simulink model "StateEstimatorComplete"  (R2022a)
settings: Solver=ode4  StartTime=0.0  StopTime=200  FixedStep=0.1  RelTol=1e-3
values from neighbouring files (symbols this model uses):
  A = [1.0034,0.0207,0.4737,0.0463,-0.2364,2.3069;    -0.0011,0.9997,-0.0541,0.1380,0.9540,-13.3772;     0.0000,0.0000,0.9424,0.6183,-0.2177,2.1255;    -0.0000,-0.0000,0.1676,-0.8000,0.4213,-5.1737;     0.0000,-0.0002,-0.0060,0.1014,-0.1223,-12.4611;    -0.0000,0.0000,-0.0000,-0.0004,-0.0028,-0.5637]    [Kalman_initializing.m]
  B = 1.0e-08 *[-0.8484,-0.3258,-0.1868;     0.4781,-0.1277,-0.2667;    -0.0948,-0.0255,-0.0254;     0.2341,0.0767,0.1066;    -0.0197,-0.0031,-0.1006;    -0.0005,-0.0006,0.0006]    [Kalman_initializing.m]
  C = [0.6830,-0.1854,-0.2271,0.6690,0.0090,0.0006 ... (first row only)    [Kalman_initializing.m]
  D = 1.0e-08 *[-0.3458,-0.1652,-0.0717;    -0.0376,-0.0129,-0.1373;     0.0011,0.0020,-0.0003]    [Kalman_initializing.m]
  K = [34.8690,9.8057,11.2373;   -20.4980,36.9942,21.6928;     4.6280,-0.6726,-33.1105;   -12.2170,-0.1861,-5.2135;    -3.8993,12.7559,16.9157;     0.0335,-0.0487,-11.0087]    [Kalman_initializing.m]
libraries: dspsrcs4 x3, realtime_pacer_lib x1
settings Model: Creator=Jan-Robin  LastModifiedBy=Jan-Robin

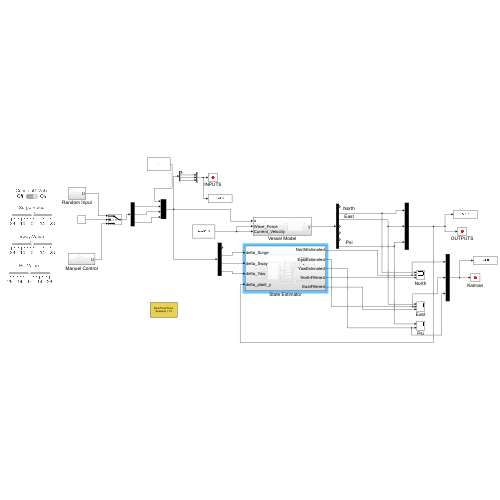
[thumbnail: Simulink's stored preview of the top-level diagram]
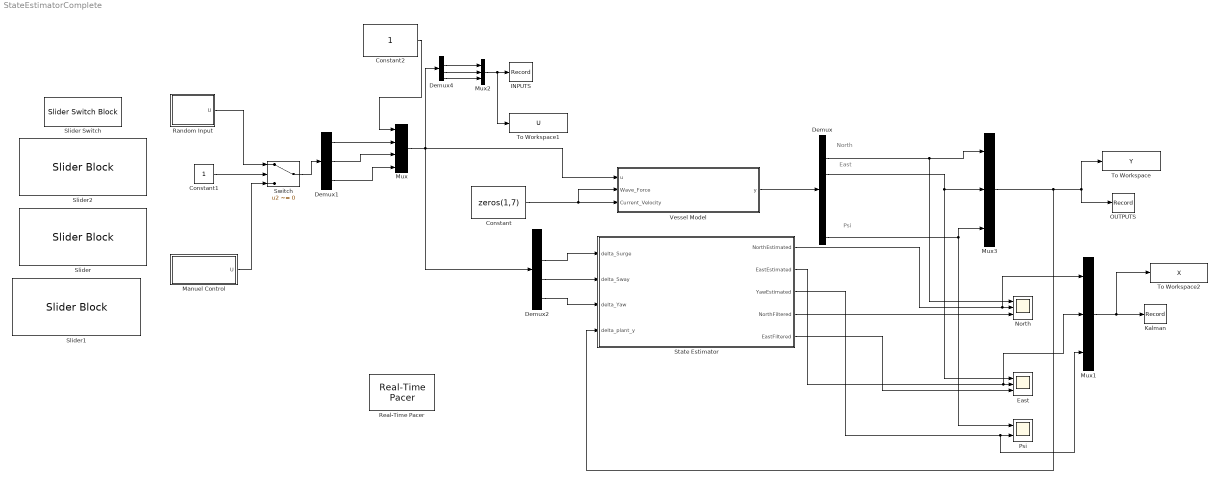
== system StateEstimatorComplete ==
  note: Psi
  note: East
  note: North
  Constant : Constant  Value=zeros(1,7)
  Constant1 : Constant
  Constant2 : Constant
  Demux : Demux  Outputs=7
  Demux1 : Demux  Outputs=3
  Demux2 : Demux
  Demux4 : Demux
  East : Scope  NumInputPorts=3
  INPUTS : Record  VariableName=INPUT  RecordToWorkspace=on  FileSettingsInternal="{\"entries\":[{\"content\":{\"excelSettings\":{\"content\":{},\"type\":\"Streamout.ExcelSettings\"}},\"type\":\"Streamout.FileSettingStorage\",\"uuid\":\"\"}],\"packageUris\":[\"http:\\/\\/schema.mathworks.com\\/mf0\\/streamout_blocks\\/R2020a\"],\"version\":\"1.0\"}"  SignalsInternal="{\"entries\":[{\"content\":{\"signals\":[{\"content\":{\"blockPath\":[],\"channel\":[],\"dimensions\":[3],\"domain\":\"\",\"hasChildren\":true,\"lineColor\":\"#ff6929\",\"plots\":[],\"port\":1,\"sid\":[\"\"],\"signalID\":6521,\"signalName\":\"Mux2\"},\"type\":\"RecordBlkView.Signal\",\"uuid\":\"\"},{\"content\":{\"blockPath\":[],\"channel\":[1],\"dimensions\":[3],\"domain\":\"\",\"lineColor\":\"#ff6929\",\"parentID\":6521,\"plots\":[1],\"port\":1,\"sid\":[\"\"],\"signalID\":6522,\"signalName\":\"Mux2\"},\"type\":\"RecordBlkView.Signal\",\"uuid\":\"\"},{\"content\":{\"blockPath\":[],\"channel\":[2],\"dimensions\":[3],\"domain\":\"\",\"lineColor\":\"#b746ff\",\"parentID\":6521,\"plots\":[1],\"port\":1,\"sid\":[\"\"],\"signalID\":6588,\"signalName\":\"Mux2\"},\"type\":\"RecordBlkView.Signal\",\"uuid\":\"\"},{\"content\":{\"blockPath\":[],\"channel\":[3],\"dimensions\":[3],\"domain\":\"\",\"lineColor\":\"#64d413\",\"parentID\":6521,\"plots\":[1],\"port\":1,\"sid\":[\"\"],\"signalID\":6589,\"signalName\":\"Mux2\"},\"type\":\"RecordBlkView.Signal\",\"uuid\":\"\"}]},\"type\":\"RecordBlkView.InputSignals\",\"uuid\":\"\"}],\"packageUris\":[\"http:\\/\\/schema.mathworks.com\\/mf0\\/streamout_blocks\\/R2020a\"],\"version\":\"1.0\"}"  VisualizationBindings="{\"sparklinesplugin\":{\"info\":[{\"bindingParametersList\":[],\"subplotID\":1}]}}"
  Kalman : Record  VariableName=KALMAN  RecordToWorkspace=on  FileSettingsInternal="{\"entries\":[{\"content\":{\"excelSettings\":{\"content\":{},\"type\":\"Streamout.ExcelSettings\"}},\"type\":\"Streamout.FileSettingStorage\",\"uuid\":\"\"}],\"packageUris\":[\"http:\\/\\/schema.mathworks.com\\/mf0\\/streamout_blocks\\/R2020a\"],\"version\":\"1.0\"}"  Layout=[1 1]  SignalsInternal="{\"entries\":[{\"content\":{\"signals\":[{\"content\":{\"blockPath\":[],\"channel\":[],\"dimensions\":[3],\"domain\":\"\",\"hasChildren\":true,\"lineColor\":\"#64d413\",\"plots\":[],\"port\":1,\"sid\":[\"\"],\"signalID\":6526,\"signalName\":\"Mux1\"},\"type\":\"RecordBlkView.Signal\",\"uuid\":\"\"},{\"content\":{\"blockPath\":[],\"channel\":[1],\"dimensions\":[3],\"domain\":\"\",\"lineColor\":\"#139fff\",\"parentID\":6526,\"plots\":[],\"port\":1,\"sid\":[\"\"],\"signalID\":6527,\"signalName\":\"Mux1\"},\"type\":\"RecordBlkView.Signal\",\"uuid\":\"\"},{\"content\":{\"blockPath\":[],\"channel\":[2],\"dimensions\":[3],\"domain\":\"\",\"lineColor\":\"#7e2f8e\",\"parentID\":6526,\"plots\":[],\"port\":1,\"sid\":[\"\"],\"signalID\":6590,\"signalName\":\"Mux1\"},\"type\":\"RecordBlkView.Signal\",\"uuid\":\"\"},{\"content\":{\"blockPath\":[],\"channel\":[3],\"dimensions\":[3],\"domain\":\"\",\"lineColor\":\"#77ac30\",\"parentID\":6526,\"plots\":[],\"port\":1,\"sid\":[\"\"],\"signalID\":6591,\"signalName\":\"Mux1\"},\"type\":\"RecordBlkView.Signal\",\"uuid\":\"\"}]},\"type\":\"RecordBlkView.InputSignals\",\"uuid\":\"\"}],\"packageUris\":[\"http:\\/\\/schema.mathworks.com\\/mf0\\/streamout_blocks\\/R2020a\"],\"version\":\"1.0\"}"  VisualizationBindings="{\"sparklinesplugin\":{\"info\":[{\"bindingParametersList\":[],\"subplotID\":1}]}}"
  Manuel Control : Subsystem
  Mux : Mux
  Mux1 : Mux  Inputs=3
  Mux2 : Mux  Inputs=3
  Mux3 : Mux  Inputs=3
  North : Scope  NumInputPorts=3
  OUTPUTS : Record  VariableName=OUTPUT  RecordToWorkspace=on  FileSettingsInternal="{\"entries\":[{\"content\":{\"excelSettings\":{\"content\":{},\"type\":\"Streamout.ExcelSettings\"}},\"type\":\"Streamout.FileSettingStorage\",\"uuid\":\"\"}],\"packageUris\":[\"http:\\/\\/schema.mathworks.com\\/mf0\\/streamout_blocks\\/R2020a\"],\"version\":\"1.0\"}"  Layout=[1 1]  SignalsInternal="{\"entries\":[{\"content\":{\"signals\":[{\"content\":{\"blockPath\":[],\"channel\":[],\"dimensions\":[3],\"domain\":\"\",\"hasChildren\":true,\"lineColor\":\"#fe330a\",\"plots\":[],\"port\":1,\"sid\":[\"\"],\"signalID\":6531,\"signalName\":\"Mux3\"},\"type\":\"RecordBlkView.Signal\",\"uuid\":\"\"},{\"content\":{\"blockPath\":[],\"channel\":[1],\"dimensions\":[3],\"domain\":\"\",\"lineColor\":\"#b746ff\",\"parentID\":6531,\"plots\":[],\"port\":1,\"sid\":[\"\"],\"signalID\":6532,\"signalName\":\"Mux3\"},\"type\":\"RecordBlkView.Signal\",\"uuid\":\"\"},{\"content\":{\"blockPath\":[],\"channel\":[2],\"dimensions\":[3],\"domain\":\"\",\"lineColor\":\"#4dbeee\",\"parentID\":6531,\"plots\":[],\"port\":1,\"sid\":[\"\"],\"signalID\":6592,\"signalName\":\"Mux3\"},\"type\":\"RecordBlkView.Signal\",\"uuid\":\"\"},{\"content\":{\"blockPath\":[],\"channel\":[3],\"dimensions\":[3],\"domain\":\"\",\"lineColor\":\"#a2142f\",\"parentID\":6531,\"plots\":[],\"port\":1,\"sid\":[\"\"],\"signalID\":6593,\"signalName\":\"Mux3\"},\"type\":\"RecordBlkView.Signal\",\"uuid\":\"\"}]},\"type\":\"RecordBlkView.InputSignals\",\"uuid\":\"\"}],\"packageUris\":[\"http:\\/\\/schema.mathworks.com\\/mf0\\/streamout_blocks\\/R2020a\"],\"version\":\"1.0\"}"  VisualizationBindings="{\"sparklinesplugin\":{\"info\":[{\"bindingParametersList\":[],\"subplotID\":1}]}}"
  Psi : Scope  NumInputPorts=2
  Random Input : Subsystem
  Real-Time Pacer : realtime_pacer_lib/Real-Time Pacer  simTimePerRealTime=10
      settings: SourceProductName=Real-Time Pacer
  Slider : SliderBlock  ScaleMin=-28  ScaleMax=28
  Slider Switch : SliderSwitchBlock
      settings: Values={{'Off', 'On'}, [0 1]}
  Slider1 : SliderBlock  ScaleMin=-28  ScaleMax=28
  Slider2 : SliderBlock  ScaleMin=-28  ScaleMax=28
  State Estimator : Subsystem
  Switch : Switch  Criteria=u2 ~= 0  SaturateOnIntegerOverflow=off  InputSameDT=off
  To Workspace : ToWorkspace  VariableName=Y  SampleTime=0.1
  To Workspace1 : ToWorkspace  VariableName=U  SampleTime=0.1
  To Workspace2 : ToWorkspace  VariableName=X  SampleTime=0.1
  Vessel Model : Subsystem
  wires:
  Demux4/3 -> Mux2/2
  Demux4/2 -> Mux2/1
  Demux4/4 -> Mux2/3
  Constant2/1 -> Mux/1
  Vessel Model/1(y) -> Demux/1
  Mux/1 -> Demux2/1, Vessel Model/1(u), Demux4/1
  Mux2/1 -> To Workspace1/1, INPUTS/1
  Demux/7 -> Psi/1, Mux3/3
  Constant/1 -> Vessel Model/2(Wave_Force), Vessel Model/3(Current_Velocity)
  Mux3/1 -> OUTPUTS/1, To Workspace/1, State Estimator/4(delta_plant_y)
  Demux2/2 -> State Estimator/1(delta_Surge)
  Demux2/3 -> State Estimator/2(delta_Sway)
  Demux2/4 -> State Estimator/3(delta_Yaw)
  Demux/2 -> Mux3/1, North/1
  State Estimator/1(NorthEstimated) -> Mux1/1, North/2
  State Estimator/2(EastEstimated) -> Mux1/2, East/2
  State Estimator/3(YawEstimated) -> Mux1/3, Psi/2
  State Estimator/4(NorthFiltered) -> North/3
  State Estimator/5(EastFiltered) -> East/3
  Mux1/1 -> To Workspace2/1, Kalman/1
  Demux/3 -> Mux3/2, East/1
  Random Input/1(U) -> Switch/1
  Constant1/1 -> Switch/2
  Manuel Control/1(U) -> Switch/3
  Switch/1 -> Demux1/1
  Demux1/1 -> Mux/2
  Demux1/2 -> Mux/3
  Demux1/3 -> Mux/4

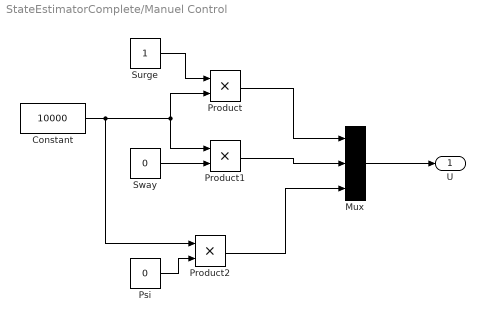
== system StateEstimatorComplete/Manuel Control ==
  Constant : Constant  Value=10000
  Mux : Mux  Inputs=3
  Product : Product
  Product1 : Product
  Product2 : Product
  Psi : Constant  Value=0
  Surge : Constant
  Sway : Constant  Value=0
  U : Outport
  wires:
  Mux/1 -> U/1
  Surge/1 -> Product/1
  Constant/1 -> Product2/1, Product/2, Product1/1
  Sway/1 -> Product1/2
  Psi/1 -> Product2/2
  Product2/1 -> Mux/3
  Product1/1 -> Mux/2
  Product/1 -> Mux/1

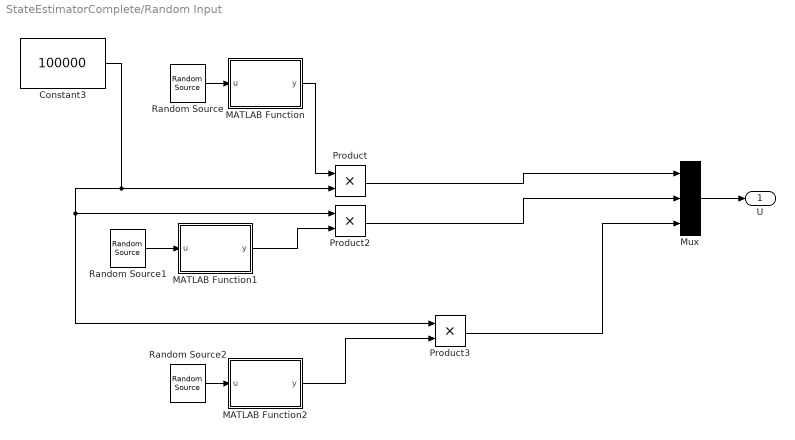
== system StateEstimatorComplete/Random Input ==
  Constant3 : Constant  Value=100000
  MATLAB Function : MATLAB Function  TreatAsAtomicUnit=on
  MATLAB Function1 : MATLAB Function  TreatAsAtomicUnit=on
  MATLAB Function2 : MATLAB Function  TreatAsAtomicUnit=on
  Mux : Mux  Inputs=3
  Product : Product
  Product2 : Product
  Product3 : Product
  Random Source : dspsrcs4/Random Source  SrcType=Uniform  NormMethod=Ziggurat  CltLength=12  MinVal=-1  MaxVal=1  MeanVal=0  VarVal=1  RepMode=Not repeatable  rawSeed=1  IsInherit=off  SampMode=Continuous  SampTime=10  SampFrame=1  DataType=Single  OutComplex=Real  OutputFrames=off
  Random Source1 : dspsrcs4/Random Source  SrcType=Uniform  NormMethod=Ziggurat  CltLength=12  MinVal=-1  MaxVal=1  MeanVal=0  VarVal=1  RepMode=Not repeatable  rawSeed=1  IsInherit=off  SampMode=Continuous  SampTime=10  SampFrame=1  DataType=Single  OutComplex=Real  OutputFrames=off
  Random Source2 : dspsrcs4/Random Source  SrcType=Uniform  NormMethod=Ziggurat  CltLength=12  MinVal=-1  MaxVal=1  MeanVal=0  VarVal=1  RepMode=Not repeatable  rawSeed=1  IsInherit=off  SampMode=Continuous  SampTime=10  SampFrame=1  DataType=Single  OutComplex=Real  OutputFrames=off
  U : Outport
  wires:
  Random Source1/1 -> MATLAB Function1/1(u)
  Constant3/1 -> Product/2, Product2/1, Product3/1
  MATLAB Function1/1(y) -> Product2/2
  Random Source2/1 -> MATLAB Function2/1(u)
  Product2/1 -> Mux/2
  Product/1 -> Mux/1
  Random Source/1 -> MATLAB Function/1(u)
  MATLAB Function2/1(y) -> Product3/2
  MATLAB Function/1(y) -> Product/1
  Product3/1 -> Mux/3
  Mux/1 -> U/1

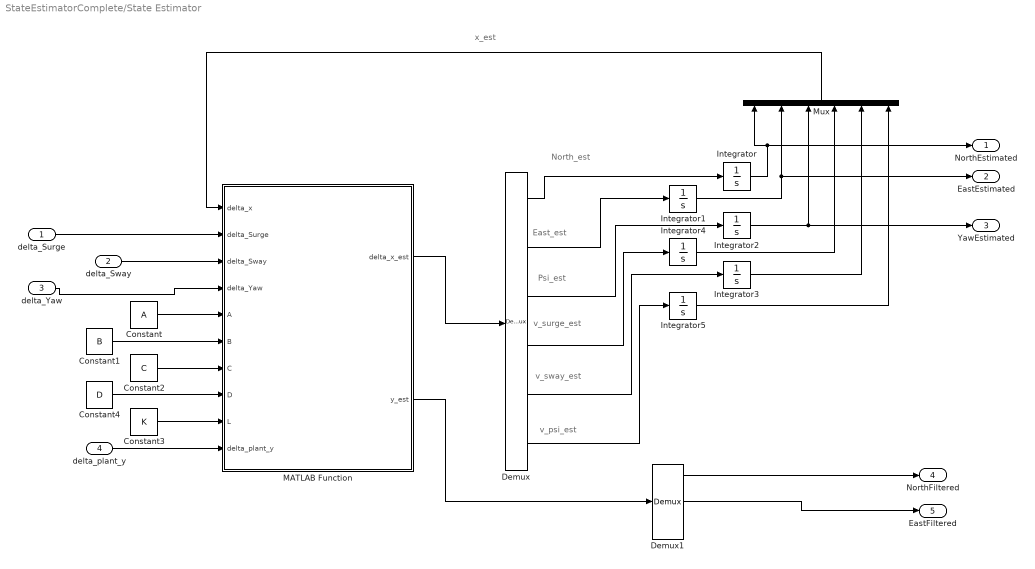
== system StateEstimatorComplete/State Estimator ==
  note: x_est
  note: v_psi_est
  note: v_sway_est
  note: v_surge_est
  note: Psi_est
  note: East_est
  note: North_est
  delta_Surge : Inport
  delta_Sway : Inport  Port=2
  delta_Yaw : Inport  Port=3
  delta_plant_y : Inport  Port=4
  Constant : Constant  Value=A
  Constant1 : Constant  Value=B
  Constant2 : Constant  Value=C
  Constant3 : Constant  Value=K
  Constant4 : Constant  Value=D
  Demux : Demux  Outputs=6
  Demux1 : Demux  Outputs=3
  Integrator : Integrator  LimitOutput=on  UpperSaturationLimit=100  LowerSaturationLimit=-100
  Integrator1 : Integrator  LimitOutput=on  UpperSaturationLimit=100  LowerSaturationLimit=-100
  Integrator2 : Integrator  InitialCondition=-0.0005  UpperSaturationLimit=0.02  LowerSaturationLimit=-0.02
  Integrator3 : Integrator  InitialCondition=0.0067  LimitOutput=on  UpperSaturationLimit=4  LowerSaturationLimit=-4
  Integrator4 : Integrator  InitialCondition=0.1385  LimitOutput=on  UpperSaturationLimit=4  LowerSaturationLimit=-4
  Integrator5 : Integrator  InitialCondition=-0.0017  LimitOutput=on  UpperSaturationLimit=0.2  LowerSaturationLimit=-0.2
  MATLAB Function : MATLAB Function  TreatAsAtomicUnit=on
  Mux : Mux  Inputs=6
  NorthEstimated : Outport
  EastEstimated : Outport  Port=2
  YawEstimated : Outport  Port=3
  NorthFiltered : Outport  Port=4
  EastFiltered : Outport  Port=5
  wires:
  delta_Surge/1 -> MATLAB Function/2(delta_Surge)
  delta_Sway/1 -> MATLAB Function/3(delta_Sway)
  delta_Yaw/1 -> MATLAB Function/4(delta_Yaw)
  delta_plant_y/1 -> MATLAB Function/10(delta_plant_y)
  Constant2/1 -> MATLAB Function/7(C)
  Constant3/1 -> MATLAB Function/9(L)
  MATLAB Function/1(delta_x_est) -> Demux/1
  Demux/1 -> Integrator/1
  Demux/2 -> Integrator1/1
  Demux/3 -> Integrator2/1
  Demux/4 -> Integrator4/1
  Demux/5 -> Integrator3/1
  Demux/6 -> Integrator5/1
  Integrator/1 -> Mux/1, NorthEstimated/1
  Integrator1/1 -> EastEstimated/1, Mux/2
  Integrator2/1 -> YawEstimated/1, Mux/3
  Integrator4/1 -> Mux/4
  Integrator3/1 -> Mux/5
  Integrator5/1 -> Mux/6
  Constant/1 -> MATLAB Function/5(A)
  Constant1/1 -> MATLAB Function/6(B)
  Constant4/1 -> MATLAB Function/8(D)
  Mux/1 -> MATLAB Function/1(delta_x)
  MATLAB Function/2(y_est) -> Demux1/1
  Demux1/1 -> NorthFiltered/1
  Demux1/2 -> EastFiltered/1

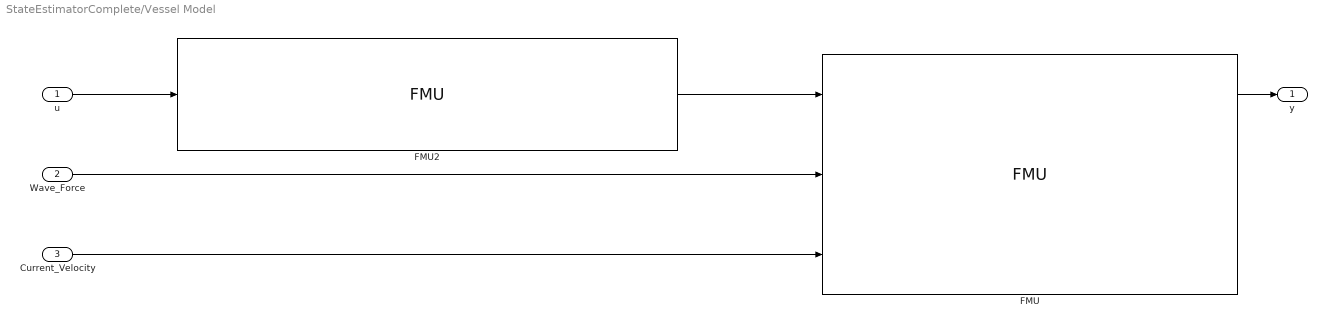
== system StateEstimatorComplete/Vessel Model ==
  u : Inport
  Wave_Force : Inport  Port=2
  Current_Velocity : Inport  Port=3
  FMU : FMU  FMUName=VesselModel.fmu  FMUMode=CoSimulation  Axc=106.0  Ayc=419.0  Bv_0_=44000.0  Bv_1_=0.0  Bv_2_=0.0  Bv_3_=0.0  Bv_4_=0.0  Bv_5_=0.0  Bv_6_=0.0  Bv_7_=177000.0  Bv_8_=0.0  Bv_9_=0.0  Bv_10_=0.0  Bv_11_=0.0  Bv_12_=0.0  Bv_13_=0.0  Bv_14_=0.0  Bv_15_=0.0  Bv_16_=0.0  Bv_17_=0.0  Bv_18_=0.0  Bv_19_=0.0  Bv_20_=0.0  Bv_21_=686000.0  Bv_22_=0.0  Bv_23_=0.0  Bv_24_=0.0  Bv_25_=0.0  Bv_26_=0.0  Bv_27_=0.0  Bv_28_=0.0  Bv_29_=0.0  Bv_30_=0.0  Bv_31_=0.0  Bv_32_=0.0  Bv_33_=0.0  Bv_34_=0.0  Bv_35_=1.0259E+7  Cx=1.0  Cy=0.7812  Dp_0_=5300.0  Dp_1_=0.0  Dp_2_=0.0  Dp_3_=0.0  Dp_4_=0.0  Dp_5_=0.0  Dp_6_=0.0  Dp_7_=21100.0  Dp_8_=0.0  Dp_9_=-20300.0  Dp_10_=0.0  Dp_11_=294000.0  Dp_12_=0.0  Dp_13_=0.0  Dp_14_=1900.0  Dp_15_=0.0  Dp_16_=-68400.0  Dp_17_=0.0  Dp_18_=0.0  Dp_19_=-20300.0  Dp_20_=0.0  Dp_21_=7600.0  Dp_22_=0.0  Dp_23_=-201300.0  Dp_24_=0.0  Dp_25_=0.0  Dp_26_=-68400.0  Dp_27_=0.0  Dp_28_=819700.0  Dp_29_=0.0  Dp_30_=0.0  Dp_31_=294000.0  Dp_32_=0.0  Dp_33_=-201300.0  Dp_34_=0.0  Dp_35_=1.8944E+6  G_0_=0.0  G_1_=0.0  G_2_=0.0  G_3_=0.0  G_4_=0.0  G_5_=0.0  G_6_=0.0  G_7_=0.0  G_8_=0.0  G_9_=0.0  G_10_=0.0  G_11_=0.0  G_12_=0.0  G_13_=0.0  G_14_=2.44E+6  G_15_=0.0  G_16_=1.78E+6  G_17_=0.0  G_18_=0.0  G_19_=0.0  G_20_=0.0  G_21_=5.11E+6  G_22_=0.0  G_23_=0.0  G_24_=0.0  G_25_=0.0  G_26_=1.78E+6  G_27_=0.0  G_28_=1.2737E+8  G_29_=0.0  G_30_=0.0  G_31_=0.0  G_32_=0.0  G_33_=0.0  G_34_=0.0  G_35_=0.0  Lpp=28.9  Minv_0_=1.268E-6  Minv_1_=0.0  Minv_2_=0.0  Minv_3_=0.0  Minv_4_=0.0  Minv_5_=0.0  Minv_6_=0.0  Minv_7_=1.083E-6  Minv_8_=0.0  Minv_9_=1.2E-8  Minv_10_=0.0  Minv_11_=1.0E-9  Minv_12_=0.0  Minv_13_=0.0  Minv_14_=5.9200000000000011E-7  Minv_15_=0.0  Minv_16_=-1.3E-8  Minv_17_=0.0  Minv_18_=0.0  Minv_19_=1.2E-8  Minv_20_=0.0  Minv_21_=1.0000000000000001E-7  Minv_22_=0.0  Minv_23_=-1.0E-9  Minv_24_=0.0  Minv_25_=0.0  Minv_26_=-1.3E-8  Minv_27_=0.0  Minv_28_=1.2E-8  Minv_29_=0.0  Minv_30_=0.0  Minv_31_=1.0E-9  Minv_32_=0.0  Minv_33_=-1.0E-9  Minv_34_=0.0  Minv_35_=2.0E-8  N=20.0  X_DOF_DP_model_Integrator1__InitialCondition_0_=0.0  X_DOF_DP_model_Integrator1__InitialCondition_1_=0.0  X_DOF_DP_model_Integrator1__InitialCondition_2_=0.0  X_DOF_DP_model_Integrator1__InitialCondition_3_=0.0  X_DOF_DP_model_Integrator1__InitialCondition_4_=0.0  X_DOF_DP_model_Integrator1__InitialCondition_5_=0.0  X_DOF_DP_model_Integrator2_InitialCondition_0_=0.0  X_DOF_DP_model_Integrator2_InitialCondition_1_=0.0  X_DOF_DP_model_Integrator2_InitialCondition_2_=0.0  X_DOF_DP_model_Integrator2_InitialCondition_3_=0.0  X_DOF_DP_model_Integrator2_InitialCondition_4_=0.0  X_DOF_DP_model_Integrator2_InitialCondition_5_=0.0  X_DOF_DP_model_Rotate_yaw_T_Constant_Value=0.0  X_DOF_DP_model_Rotate_yaw_T_psi_Value=0.0  X_DOF_DP_model_X_DOF_transformation_Euler_angles_to_att=0.0  X_DOF_DP_model_X_DOF_transformation_Euler_angles_to_att_2=1.0  X_DOF_DP_model_zero_Value=0.0  rho=1025.0  mask(VesselModel [Co-Simulation, v2.0]){}
      mask Display:
      | disp('VesselModel');
      | port_label('output',1,'Vessel_Position');
      | port_label('output',2,'Vessel_Velocity');
      | port_label('output',3,'Vessel_Acceleration');
      | port_label('input',1,'Thrust');
      | port_label('input',2,'Wave_Forces');
      | port_label('input',3,'Current_Velocity');
  FMU2 : FMU  FMUName=ThrusterDynamics.fmu  FMUMode=CoSimulation  Heave_Thrust=struct('Value',0.0)  Merge1=struct('InitialOutput',0.0)  Pitch_Thrust=struct('Value',0.0)  Roll_Thrust=struct('Value',0.0)  Thruster_Dynamics=struct('Surge_Thrust_Dynamics',struct('A',-0.2,'C',0.2),'Sway_Thrust_Dynamics',struct('A',-0.2,'C',0.2),'Yaw_Thrust_Dynamics',struct('A',-0.2,'C',0.2))  enableDynamics=on  enableSaturation=on  maxThrust=[1.0E+10,1.0E+10,1.0E+11]  mask(ThrusterDynamics [Co-Simulation, v2.0]){}
      mask Display:
      | disp('ThrusterDynamics');
      | port_label('output',1,'Thrust');
      | port_label('input',1,'Commanded_Thrust');
  y : Outport
  wires:
  u/1 -> FMU2/1
  FMU2/1 -> FMU/1
  FMU/1 -> y/1
  Wave_Force/1 -> FMU/2
  Current_Velocity/1 -> FMU/3

== matlab function StateEstimatorComplete/Random Input/MATLAB Function1 ==
  data: u input; y output
function y = fcn(u)

if (u> 0)
    y=1;

else
    y=-1;
end

== matlab function StateEstimatorComplete/Random Input/MATLAB Function ==
  data: u input; y output
function y = fcn(u)

if (u> 0)
    y=1;

else
    y=-1;
end

== matlab function StateEstimatorComplete/Random Input/MATLAB Function2 ==
  data: u input; y output
function y = fcn(u)

if (u> 0)
    y=1;

else
    y=-1;
end

== matlab function StateEstimatorComplete/State Estimator/MATLAB Function ==
  data: delta_x input; delta_x_est output; delta_Surge input; delta_Sway input; delta_Yaw input; A input; B input; C input; D input; L input; delta_plant_y input; y_est output
function [delta_x_est,y_est]= state_estimator(delta_x, delta_Surge, delta_Sway, delta_Yaw,A, B,C, D,L,delta_plant_y)

y_est = C*delta_x+D*[delta_Surge;delta_Sway;delta_Yaw];
delta_x_est = A*delta_x +B*[delta_Surge;delta_Sway;delta_Yaw] + L*(delta_plant_y-y_est);
